simulink model "eAgriBot_V4"  (R2022b)
settings: Solver=ode3  StartTime=0.0  StopTime=t_sim  FixedStep=step_size  RelTol=1e-3
values from neighbouring files (symbols this model uses):
  accel = 0.1*9.81    (= 0.981)    [Run_eAgriBot_V4.m]
  B_tines = 5    [Run_eAgriBot_V4.m]
  brake_bias = 1    [Run_eAgriBot_V4.m]
  c = 6100    [Run_eAgriBot_V4.m]
  decel = 0.15*9.81    (= 1.4715)    [Run_eAgriBot_V4.m]
  decel_begin_dist = total_dist_target    (= 100)    [Run_eAgriBot_V4.m]
  drivetype = 3    [Run_eAgriBot_V4.m]
  effmap = [0.5 0.586 0.723 0.778 0.614 0.604 0.6 0.584 0.709 0.658 0.586 0.688 ... (121 elements, 11x11)]    [EM_effmap_generic.mat]
  end_delay = 4    [Run_eAgriBot_V4.m]
  F_tines = 5    [Run_eAgriBot_V4.m]
  Fb_max = m*g    (= 5101.2)    [Run_eAgriBot_V4.m]
  FT_c_x_rel = l_f    (= 0.645)    [Run_eAgriBot_V4.m]
  FT_c_z_rel = R_u-h_CoG    (= -0.2825)    [Run_eAgriBot_V4.m]
  g = 9.81    [Run_eAgriBot_V4.m]
  gb_eff = 0.98    [Run_eAgriBot_V4.m]
  ground_coh = c*ones(length(ground_points),1)    [Run_eAgriBot_V4.m]
  ground_dens = gamma_s*ones(length(ground_points),1)    [Run_eAgriBot_V4.m]
  ground_height = zeros(length(ground_points),1)    [Run_eAgriBot_V4.m]
  ground_kxy = k_xy*ones(length(ground_points),1)    [Run_eAgriBot_V4.m]
  ground_res = 0.01    [Run_eAgriBot_V4.m]
  Har_back_tip_x_rel = Har_back_top_x_rel+Har_tine_length*cos(Har_angle)    [Run_eAgriBot_V4.m]
  Har_back_tip_z_rel = abs(Hook_z_rel)-h_CoG-Har_tine_depth    [Run_eAgriBot_V4.m]
  Har_back_top_x_rel = -2.0    (= -2)    [Run_eAgriBot_V4.m]
  Har_back_top_z_rel = Har_back_tip_z_rel+Har_tine_length*sin(Har_angle)    [Run_eAgriBot_V4.m]
  Har_front_tip_x_rel = Har_front_top_x_rel+Har_tine_length*cos(Har_angle)    [Run_eAgriBot_V4.m]
  Har_front_tip_z_rel = abs(Hook_z_rel)-h_CoG-Har_tine_depth    [Run_eAgriBot_V4.m]
  Har_front_top_x_rel = -1.2    [Run_eAgriBot_V4.m]
  Har_front_top_z_rel = Har_front_tip_z_rel+Har_tine_length*sin(Har_angle)    [Run_eAgriBot_V4.m]
  Har_tine_length = 0.25    [Run_eAgriBot_V4.m]
  Har_tine_width = 0.02    [Run_eAgriBot_V4.m]
  Har_tire_rad = 0.5842/2    (= 0.2921)    [Run_eAgriBot_V4.m]
  Har_tire_x_rel = -1.5    [Run_eAgriBot_V4.m]
  Har_tire_z_rel = abs(Hook_z_rel)-h_CoG+Har_tire_rad    [Run_eAgriBot_V4.m]
  Hook_x_rel = l_f-l-0.4    (= -1.045)    [Run_eAgriBot_V4.m]
  Hook_z_rel = -0.3    [Run_eAgriBot_V4.m]
  i_front = 17.9542    [Run_eAgriBot_V4.m]
  I_gain = 0.0    (= 0)    [Run_eAgriBot_V4.m]
  i_rear = 17.9542    [Run_eAgriBot_V4.m]
  I_y = 150    [Run_eAgriBot_V4.m]
  I_y_tool = 20    [Run_eAgriBot_V4.m]
  index_init = round(FT_init_exit_x/ground_res)+1    [Run_eAgriBot_V4.m]
  init_CoG_height = h_CoG-0.001    (= 0.599)    [Run_eAgriBot_V4.m]
  init_CoG_v_z = 0    [Run_eAgriBot_V4.m]
  init_omega = 0    [Run_eAgriBot_V4.m]
  init_theta = 0    [Run_eAgriBot_V4.m]
  J_front = J_drive    (= 15)    [Run_eAgriBot_V4.m]
  J_harrow = 1    [Run_eAgriBot_V4.m]
  J_rear = J_drive    (= 15)    [Run_eAgriBot_V4.m]
  k_d = 50e2    (= 5000)    [Run_eAgriBot_V4.m]
  k_d_har = 50e2    (= 5000)    [Run_eAgriBot_V4.m]
  m = 520    [Run_eAgriBot_V4.m]
  m_tool = 200    [Run_eAgriBot_V4.m]
  main_cycle_delay = 5    [Run_eAgriBot_V4.m]
  mu = 0.35    [Run_eAgriBot_V4.m]
  omega_tool_init = 0    [Run_eAgriBot_V4.m]
  P_aux = 200    [Run_eAgriBot_V4.m]
  P_gain = 1.0    (= 1)    [Run_eAgriBot_V4.m]
  pack_Ah = 360    [Battery_data_V5_Kokam_NMC.mat]
  pack_R_charge = [0.00267222222222 0.00267222222222 0.00317777777778 0.00310555555556 0.0026 0.00281666666667 0.00332222222222 0.00353888888889 0.00325 0.00382777777778 0.00382777777778]    [Battery_data_V5_Kokam_NMC.mat]
  pack_R_discharge = [0.00267222222222 0.00267222222222 0.00317777777778 0.00310555555556 0.0026 0.00281666666667 0.00332222222222 0.00353888888889 0.00325 0.00382777777778 0.00382777777778]    [Battery_data_V5_Kokam_NMC.mat]
  pack_VOC = [54.509 52.351 50.895 49.556 48.477 47.645 47.008 46.449 45.825 44.941 44.941]    [Battery_data_V5_Kokam_NMC.mat]
  params2 = [exit_angle reso theta_m_max s_d_tol po]    [Run_eAgriBot_V4.m]
  phi = 26.6    [Run_eAgriBot_V4.m]
  pre_accel = 0.1*9.81    (= 0.981)    [Run_eAgriBot_V4.m]
  pre_decel = 0.15*9.81    (= 1.4715)    [Run_eAgriBot_V4.m]
  pre_decel_begin_dist = pre_dist_target-pre_decel_dist    (= 2.34454218631)    [Run_eAgriBot_V4.m]
  pre_vel = 5    [Run_eAgriBot_V4.m]
  r_front = R_u    (= 0.3175)    [Run_eAgriBot_V4.m]
  r_rear = R_u    (= 0.3175)    [Run_eAgriBot_V4.m]
  rho_t = gamma_s/9.81    (= 1664.01630989)    [Run_eAgriBot_V4.m]
  RT_c_x_rel = l_f-l    (= -0.645)    [Run_eAgriBot_V4.m]
  RT_c_z_rel = R_u-h_CoG    (= -0.2825)    [Run_eAgriBot_V4.m]
  s_init = 3    [Run_eAgriBot_V4.m]
  simu_max_time = cycle_total_time*4    (= 259.930519878)    [Run_eAgriBot_V4.m]
  slip_init = 0    [Run_eAgriBot_V4.m]
  slip_ub = r_rear*1.75    (= 0.555625)    [Run_eAgriBot_V4.m]
  slip_ub_har = Har_tire_rad*1.90    (= 0.55499)    [Run_eAgriBot_V4.m]
  SOC_init = 0.8    [Run_eAgriBot_V4.m]
  SOD = [0 0.1 0.2 0.3 0.4 0.5 0.6 0.7 0.8 0.9 1]    [Battery_data_V5_Kokam_NMC.mat]
  sr_lim_skid = -0.2    [Run_eAgriBot_V4.m]
  sr_lim_slip_f = 0.20-slip_trig    (= 0.18)    [Run_eAgriBot_V4.m]
  sr_lim_slip_r = 0.14-slip_trig    (= 0.12)    [Run_eAgriBot_V4.m]
  step_size = 1e-3    (= 0.001)    [Run_eAgriBot_V4.m]
  T = [80 80 75 70.5882352941 66.6666666667 63.1578947368 60 57.1428571429 54.5454545455 52.1739130435 50 48 ... (49 elements, 49x1)]    [EM_data_V4.mat]    (also in Run_eAgriBot_V4.m = 2*T)
  T_effmap = [0 8 16 24 32 40 48 56 64 72 80]    [EM_effmap_generic.mat]    (also in Run_eAgriBot_V4.m = 2*T_effmap)
  T_multi_r = 1.5    [Run_eAgriBot_V4.m]
  t_params = [c k_c k_phi phi k_xy gamma_s R_u wid c_0 c_1 c_0f c_1f n_0 n_1 k_1 k_2 k_3]    [Run_eAgriBot_V4.m]
  t_params_har = [c k_c k_phi phi k_xy gamma_s Har_tire_rad Har_tire_wid c_0 c_1 c_0f c_1f n_0 n_1 k_1 k_2 k_3]    [Run_eAgriBot_V4.m]
  theta_tool_init = 0    [Run_eAgriBot_V4.m]
  Tine_vz_damping = 0    [Run_eAgriBot_V4.m]
  Tool_x_rel = -1.3    [Run_eAgriBot_V4.m]
  Tool_z_rel = -0.08    [Run_eAgriBot_V4.m]
  v_init = 0    [Run_eAgriBot_V4.m]
  vel_max = 8    [Run_eAgriBot_V4.m]
  w = [0 75 80 85 90 95 100 105 110 115 120 125 ... (49 elements, 49x1)]    [EM_data_V4.mat]
  w_effmap = [0 31.4159265359 62.8318530718 94.2477796077 125.663706144 157.079632679 188.495559215 219.911485751 251.327412287 282.743338823 314.159265359]    [EM_effmap_generic.mat]
libraries: slpidlib x1, simulink x1
(part 2 of 4)

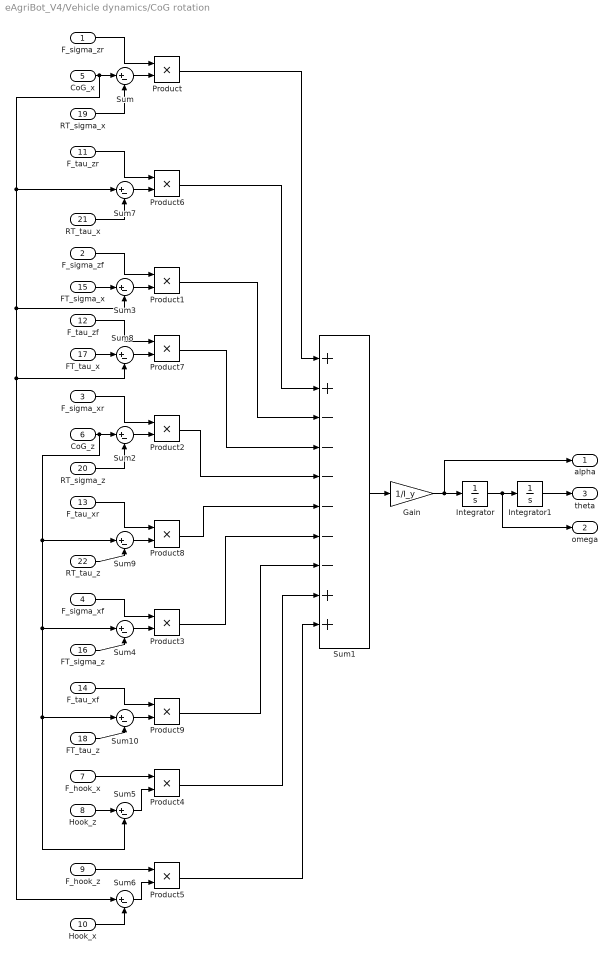
== system eAgriBot_V4/Vehicle dynamics/CoG rotation ==
  F_sigma_zr : Inport
  F_sigma_zf : Inport  Port=2
  F_sigma_xr : Inport  Port=3
  F_sigma_xf : Inport  Port=4
  CoG_x : Inport  Port=5
  CoG_z : Inport  Port=6
  F_hook_x : Inport  Port=7
  Hook_z : Inport  Port=8
  F_hook_z : Inport  Port=9
  Hook_x : Inport  Port=10
  F_tau_zr : Inport  Port=11
  F_tau_zf : Inport  Port=12
  F_tau_xr : Inport  Port=13
  F_tau_xf : Inport  Port=14
  FT_sigma_x : Inport  Port=15
  FT_sigma_z : Inport  Port=16
  FT_tau_x : Inport  Port=17
  FT_tau_z : Inport  Port=18
  RT_sigma_x : Inport  Port=19
  RT_sigma_z : Inport  Port=20
  RT_tau_x : Inport  Port=21
  RT_tau_z : Inport  Port=22
  Gain : Gain  Gain=1/I_y
  Integrator : Integrator  InitialCondition=init_omega
  Integrator1 : Integrator  InitialCondition=init_theta
  Product{,1..9} (10 alike) : Product
  Sum{,2..10} (10 alike) : Sum  Inputs=|+-
  Sum1 : Sum  Inputs=++------++
  alpha : Outport
  omega : Outport  Port=2
  theta : Outport  Port=3
  wires:
  Sum/1 -> Product/2
  F_sigma_zr/1 -> Product/1
  Product/1 -> Sum1/1
  RT_sigma_x/1 -> Sum/2
  Sum3/1 -> Product1/2
  FT_sigma_x/1 -> Sum3/1
  F_sigma_zf/1 -> Product1/1
  Sum1/1 -> Gain/1
  Integrator/1 -> omega/1, Integrator1/1
  Integrator1/1 -> theta/1
  F_sigma_xr/1 -> Product2/1
  Sum2/1 -> Product2/2
  RT_sigma_z/1 -> Sum2/2
  F_sigma_xf/1 -> Product3/1
  Sum4/1 -> Product3/2
  FT_sigma_z/1 -> Sum4/2
  Gain/1 -> alpha/1, Integrator/1
  F_hook_x/1 -> Product4/1
  Hook_z/1 -> Sum5/1
  Sum5/1 -> Product4/2
  F_hook_z/1 -> Product5/1
  Sum6/1 -> Product5/2
  Hook_x/1 -> Sum6/2
  CoG_x/1 -> Sum/1, Sum7/1, Sum6/1, Sum8/2, Sum3/2
  F_tau_zr/1 -> Product6/1
  RT_tau_x/1 -> Sum7/2
  Sum7/1 -> Product6/2
  Product1/1 -> Sum1/3
  Product6/1 -> Sum1/2
  Product2/1 -> Sum1/5
  Sum8/1 -> Product7/2
  F_tau_zf/1 -> Product7/1
  FT_tau_x/1 -> Sum8/1
  Product7/1 -> Sum1/4
  RT_tau_z/1 -> Sum9/2
  Sum9/1 -> Product8/2
  F_tau_xr/1 -> Product8/1
  CoG_z/1 -> Sum2/1, Sum9/1, Sum10/1, Sum5/2, Sum4/1
  Product3/1 -> Sum1/7
  Product8/1 -> Sum1/6
  FT_tau_z/1 -> Sum10/2
  Sum10/1 -> Product9/2
  F_tau_xf/1 -> Product9/1
  Product4/1 -> Sum1/9
  Product5/1 -> Sum1/10
  Product9/1 -> Sum1/8

== system eAgriBot_V4/Vehicle dynamics/Ground properties update for rear tire ==
  FT_x : Inport
  FT_z : Inport  Port=2
  sr_f : Inport  Port=3
  RT_x : Inport  Port=4
  RT_z : Inport  Port=5
  Constant : Constant  Value=ground_res
  Constant1 : Constant  Value=ground_res
  Constant2 : Constant  Value=params2
  Constant3 : Constant  Value=t_params
  Constant4 : Constant  Value=t_params
  Delay : Delay  DelayLength=1  InitialCondition=ground_height  SampleTime=step_size
  Delay1 : Delay  DelayLength=1  InitialCondition=index_init  SampleTime=step_size
  Delay2 : Delay  DelayLength=1  InitialCondition=ground_kxy  SampleTime=step_size
  Delay3 : Delay  DelayLength=1  InitialCondition=ground_coh  SampleTime=step_size
  Delay4 : Delay  DelayLength=1  InitialCondition=ground_dens  SampleTime=step_size
  MATLAB Function : MATLAB Function  TreatAsAtomicUnit=on  SystemSampleTime=step_size
  MATLAB Function1 : MATLAB Function  TreatAsAtomicUnit=on  SystemSampleTime=step_size
  Mux : Mux
  To Workspace : ToWorkspace  VariableName=new_gh  SampleTime=step_size
      settings: MaxDataPoints=1  Save2DSignal=2-D array (concatenate along first dimension)
  To Workspace1 : ToWorkspace  VariableName=new_dens  SampleTime=step_size
      settings: MaxDataPoints=1
  To Workspace2 : ToWorkspace  VariableName=new_coh  SampleTime=step_size
      settings: MaxDataPoints=1
  To Workspace3 : ToWorkspace  VariableName=new_kx  SampleTime=step_size
      settings: MaxDataPoints=1
  To Workspace4 : ToWorkspace  VariableName=RT_z_relative  SaveFormat=Timeseries  SampleTime=step_size
  RT_upd_params : Outport
  index_upd_high : Outport  Port=2
  index_upd_low : Outport  Port=3
  upd_h : Outport  Port=4
  upd_rho : Outport  Port=5
  upd_coh : Outport  Port=6
  upd_kx : Outport  Port=7
  wires:
  Constant/1 -> MATLAB Function/2(ground_res)
  FT_x/1 -> MATLAB Function/4(FT_x)
  FT_z/1 -> MATLAB Function/5(FT_z)
  Constant2/1 -> MATLAB Function/3(params2)
  MATLAB Function/3(ground_height) -> upd_h/1, Delay/1, To Workspace/1
  MATLAB Function/7(index) -> Delay1/1
  Delay/1 -> MATLAB Function/7("ground_height "), MATLAB Function1/3(ground_height)
  Delay1/1 -> MATLAB Function/11(prev_index)
  Constant3/1 -> MATLAB Function/1(t_params)
  sr_f/1 -> MATLAB Function/6(sr_f)
  MATLAB Function/6(kx) -> upd_kx/1, Delay2/1, To Workspace3/1
  Delay2/1 -> MATLAB Function/10("kx "), MATLAB Function1/6(kx)
  MATLAB Function/5(coh) -> upd_coh/1, Delay3/1, To Workspace2/1
  Delay3/1 -> MATLAB Function/9("coh "), MATLAB Function1/5(coh)
  MATLAB Function/4(dens) -> upd_rho/1, Delay4/1, To Workspace1/1
  Delay4/1 -> MATLAB Function/8("dens "), MATLAB Function1/4(dens)
  RT_x/1 -> MATLAB Function1/1(RT_x)
  Constant1/1 -> MATLAB Function1/7(ground_res)
  Constant4/1 -> MATLAB Function1/8(t_params)
  RT_z/1 -> MATLAB Function1/2(RT_z)
  MATLAB Function1/1(upd_RT_z) -> To Workspace4/1, Mux/1
  MATLAB Function1/2(upd_dens) -> Mux/2
  MATLAB Function1/3(upd_coh) -> Mux/3
  MATLAB Function1/4(upd_kx) -> Mux/4
  Mux/1 -> RT_upd_params/1
  MATLAB Function/1(index_upd_high) -> index_upd_high/1
  MATLAB Function/2(index_upd_low) -> index_upd_low/1

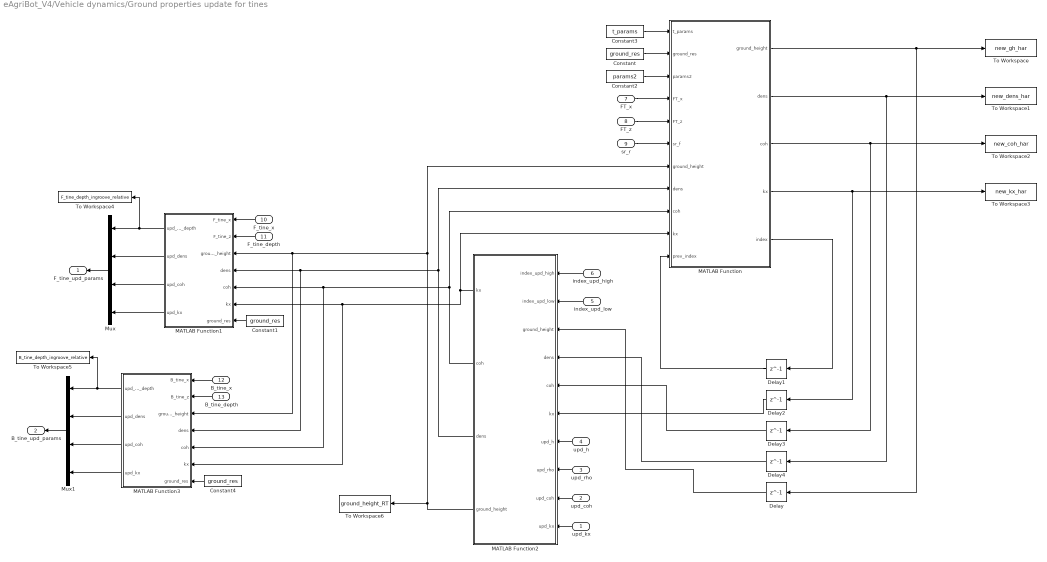
== system eAgriBot_V4/Vehicle dynamics/Ground properties update for tines ==
  upd_kx : Inport
  upd_coh : Inport  Port=2
  upd_rho : Inport  Port=3
  upd_h : Inport  Port=4
  index_upd_low : Inport  Port=5
  index_upd_high : Inport  Port=6
  FT_x : Inport  Port=7
  FT_z : Inport  Port=8
  sr_r : Inport  Port=9
  F_tine_x : Inport  Port=10
  F_tine_depth : Inport  Port=11
  B_tine_x : Inport  Port=12
  B_tine_depth : Inport  Port=13
  Constant : Constant  Value=ground_res
  Constant1 : Constant  Value=ground_res
  Constant2 : Constant  Value=params2
  Constant3 : Constant  Value=t_params
  Constant4 : Constant  Value=ground_res
  Delay : Delay  DelayLength=1  InitialCondition=ground_height  SampleTime=step_size
  Delay1 : Delay  DelayLength=1  InitialCondition=index_init  SampleTime=step_size
  Delay2 : Delay  DelayLength=1  InitialCondition=ground_kxy  SampleTime=step_size
  Delay3 : Delay  DelayLength=1  InitialCondition=ground_coh  SampleTime=step_size
  Delay4 : Delay  DelayLength=1  InitialCondition=ground_dens  SampleTime=step_size
  MATLAB Function : MATLAB Function  TreatAsAtomicUnit=on  SystemSampleTime=step_size
  MATLAB Function1 : MATLAB Function  TreatAsAtomicUnit=on  SystemSampleTime=step_size
  MATLAB Function2 : MATLAB Function  TreatAsAtomicUnit=on  SystemSampleTime=step_size
  MATLAB Function3 : MATLAB Function  TreatAsAtomicUnit=on  SystemSampleTime=step_size
  Mux : Mux
  Mux1 : Mux
  To Workspace : ToWorkspace  VariableName=new_gh_har  SampleTime=step_size
      settings: MaxDataPoints=1  Save2DSignal=2-D array (concatenate along first dimension)
  To Workspace1 : ToWorkspace  VariableName=new_dens_har  SampleTime=step_size
      settings: MaxDataPoints=1
  To Workspace2 : ToWorkspace  VariableName=new_coh_har  SampleTime=step_size
      settings: MaxDataPoints=1
  To Workspace3 : ToWorkspace  VariableName=new_kx_har  SampleTime=step_size
      settings: MaxDataPoints=1
  To Workspace4 : ToWorkspace  VariableName=F_tine_depth_ingroove_relative  SaveFormat=Timeseries  SampleTime=step_size
  To Workspace5 : ToWorkspace  VariableName=B_tine_depth_ingroove_relative  SaveFormat=Timeseries  SampleTime=step_size
  To Workspace6 : ToWorkspace  VariableName=ground_height_RT  SampleTime=-1
      settings: MaxDataPoints=1
  F_tine_upd_params : Outport
  B_tine_upd_params : Outport  Port=2
  wires:
  Constant/1 -> MATLAB Function/2(ground_res)
  FT_x/1 -> MATLAB Function/4(FT_x)
  FT_z/1 -> MATLAB Function/5(FT_z)
  Constant2/1 -> MATLAB Function/3(params2)
  MATLAB Function/1(ground_height) -> Delay/1, To Workspace/1
  MATLAB Function/5(index) -> Delay1/1
  Delay/1 -> MATLAB Function2/3("ground_height ")
  Delay1/1 -> MATLAB Function/11(prev_index)
  Constant3/1 -> MATLAB Function/1(t_params)
  sr_r/1 -> MATLAB Function/6(sr_f)
  MATLAB Function/4(kx) -> To Workspace3/1, Delay2/1
  Delay2/1 -> MATLAB Function2/6("kx ")
  MATLAB Function/3(coh) -> To Workspace2/1, Delay3/1
  Delay3/1 -> MATLAB Function2/5("coh ")
  MATLAB Function/2(dens) -> To Workspace1/1, Delay4/1
  Delay4/1 -> MATLAB Function2/4("dens ")
  F_tine_x/1 -> MATLAB Function1/1(F_tine_x)
  Constant1/1 -> MATLAB Function1/7(ground_res)
  F_tine_depth/1 -> MATLAB Function1/2(F_tine_z)
  MATLAB Function1/1(upd_F_tine_depth) -> To Workspace4/1, Mux/1
  MATLAB Function1/2(upd_dens) -> Mux/2
  MATLAB Function1/3(upd_coh) -> Mux/3
  MATLAB Function1/4(upd_kx) -> Mux/4
  Mux/1 -> F_tine_upd_params/1
  index_upd_high/1 -> MATLAB Function2/1(index_upd_high)
  index_upd_low/1 -> MATLAB Function2/2(index_upd_low)
  MATLAB Function2/4(ground_height) -> To Workspace6/1, MATLAB Function/7("ground_height "), MATLAB Function3/3(ground_height), MATLAB Function1/3(ground_height)
  MATLAB Function2/3(dens) -> MATLAB Function/8("dens "), MATLAB Function3/4(dens), MATLAB Function1/4(dens)
  MATLAB Function2/2(coh) -> MATLAB Function/9("coh "), MATLAB Function3/5(coh), MATLAB Function1/5(coh)
  MATLAB Function2/1(kx) -> MATLAB Function3/6(kx), MATLAB Function1/6(kx), MATLAB Function/10("kx ")
  Constant4/1 -> MATLAB Function3/7(ground_res)
  MATLAB Function3/1(upd_B_tine_depth) -> To Workspace5/1, Mux1/1
  Mux1/1 -> B_tine_upd_params/1
  MATLAB Function3/4(upd_kx) -> Mux1/4
  B_tine_depth/1 -> MATLAB Function3/2(B_tine_z)
  B_tine_x/1 -> MATLAB Function3/1(B_tine_x)
  MATLAB Function3/2(upd_dens) -> Mux1/2
  MATLAB Function3/3(upd_coh) -> Mux1/3
  upd_h/1 -> MATLAB Function2/7(upd_h)
  upd_rho/1 -> MATLAB Function2/8(upd_rho)
  upd_coh/1 -> MATLAB Function2/9(upd_coh)
  upd_kx/1 -> MATLAB Function2/10(upd_kx)

== system eAgriBot_V4/Vehicle dynamics/Position and velocity of the wheels (output values are for wheel bottom points) ==
  theta : Inport
  omega : Inport  Port=2
  CoG_vx : Inport  Port=3
  CoG_x : Inport  Port=4
  CoG_vz : Inport  Port=5
  CoG_z : Inport  Port=6
  F_sigma_anglef : Inport  Port=7
  F_tau_anglef : Inport  Port=8
  F_sigma_angler : Inport  Port=9
  F_tau_angler : Inport  Port=10
  Constant : Constant  Value=RT_c_z_rel
  Constant1 : Constant  Value=RT_c_x_rel
  Constant2 : Constant  Value=FT_c_z_rel
  Constant3 : Constant  Value=FT_c_x_rel
  Constant4 : Constant  Value=r_rear
  Constant5 : Constant  Value=r_front
  MATLAB Function : MATLAB Function  TreatAsAtomicUnit=on  SystemSampleTime=step_size
  MATLAB Function1 : MATLAB Function  TreatAsAtomicUnit=on  SystemSampleTime=step_size
  RT_x : Outport
  RT_z : Outport  Port=2
  FT_x : Outport  Port=3
  FT_z : Outport  Port=4
  RT_vx : Outport  Port=5
  RT_vz : Outport  Port=6
  FT_vx : Outport  Port=7
  FT_vz : Outport  Port=8
  FT_sigma_x : Outport  Port=9
  FT_sigma_z : Outport  Port=10
  FT_tau_x : Outport  Port=11
  FT_tau_z : Outport  Port=12
  RT_sigma_x : Outport  Port=13
  RT_sigma_z : Outport  Port=14
  RT_tau_x : Outport  Port=15
  RT_tau_z : Outport  Port=16
  wires:
  MATLAB Function/4(FT_z) -> MATLAB Function1/4(FT_z), FT_z/1
  MATLAB Function/8(FT_vz) -> FT_vz/1
  CoG_vz/1 -> MATLAB Function/5(CoG_vz)
  theta/1 -> MATLAB Function/1(theta)
  CoG_vx/1 -> MATLAB Function/3(CoG_vx)
  MATLAB Function/1(RT_x) -> MATLAB Function1/1(RT_x), RT_x/1
  omega/1 -> MATLAB Function/2(omega)
  MATLAB Function/6(RT_vz) -> RT_vz/1
  MATLAB Function/3(FT_x) -> MATLAB Function1/3(FT_x), FT_x/1
  MATLAB Function/7(FT_vx) -> FT_vx/1
  MATLAB Function/5(RT_vx) -> RT_vx/1
  CoG_z/1 -> MATLAB Function/6(CoG_z)
  CoG_x/1 -> MATLAB Function/4(CoG_x)
  MATLAB Function/2(RT_z) -> MATLAB Function1/2(RT_z), RT_z/1
  Constant/1 -> MATLAB Function/7(RT_c_z_rel)
  Constant1/1 -> MATLAB Function/8(RT_c_x_rel)
  Constant2/1 -> MATLAB Function/9(FT_c_z_rel)
  Constant3/1 -> MATLAB Function/10(FT_c_x_rel)
  Constant4/1 -> MATLAB Function1/5(r_rear), MATLAB Function/11(r_rear)
  Constant5/1 -> MATLAB Function/12(r_front), MATLAB Function1/6(r_front)
  MATLAB Function1/1(FT_sigma_x) -> FT_sigma_x/1
  MATLAB Function1/2(FT_sigma_z) -> FT_sigma_z/1
  MATLAB Function1/3(FT_tau_x) -> FT_tau_x/1
  MATLAB Function1/4(FT_tau_z) -> FT_tau_z/1
  MATLAB Function1/5(RT_sigma_x) -> RT_sigma_x/1
  MATLAB Function1/6(RT_sigma_z) -> RT_sigma_z/1
  MATLAB Function1/7(RT_tau_x) -> RT_tau_x/1
  MATLAB Function1/8(RT_tau_z) -> RT_tau_z/1
  F_sigma_anglef/1 -> MATLAB Function1/7(F_sigma_anglef)
  F_tau_anglef/1 -> MATLAB Function1/8(F_tau_anglef)
  F_sigma_angler/1 -> MATLAB Function1/9(F_sigma_angler)
  F_tau_angler/1 -> MATLAB Function1/10(F_tau_angler)

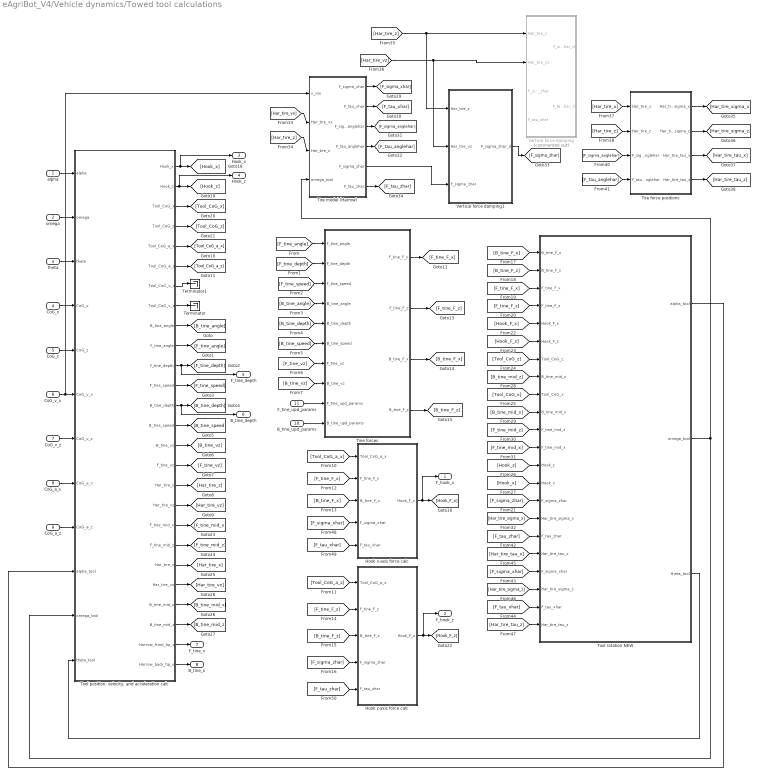
== system eAgriBot_V4/Vehicle dynamics/Towed tool calculations ==
  alpha : Inport
  omega : Inport  Port=2
  theta : Inport  Port=3
  CoG_x : Inport  Port=4
  CoG_z : Inport  Port=5
  CoG_v_x : Inport  Port=6
  CoG_v_z : Inport  Port=7
  CoG_a_x : Inport  Port=8
  CoG_a_z : Inport  Port=9
  B_tine_upd_params : Inport  Port=10
  F_tine_upd_params : Inport  Port=11
  Hook x-axis force calc : Subsystem
      settings: MinAlgLoopOccurrences=on
  Hook z-axis force calc : Subsystem
      settings: MinAlgLoopOccurrences=on
  Terminator : Terminator
  Terminator1 : Terminator
  Tine forces : Subsystem
  Tire force positions : Subsystem
  Tire model (Harrow) : Subsystem
  "Tool position, velocity, and acceleration calc" : Subsystem
      settings: MinAlgLoopOccurrences=on
  Tool rotation NEW : Subsystem
  Vertical force damping : Subsystem  Commented=on
  Vertical force damping1 : Subsystem
  F_hook_x : Outport
  F_hook_z : Outport  Port=2
  Hook_x : Outport  Port=3
  Hook_z : Outport  Port=4
  F_tine_depth : Outport  Port=5
  B_tine_depth : Outport  Port=6
  F_tine_x : Outport  Port=7
  B_tine_x : Outport  Port=8
  wires:
  alpha/1 -> "Tool position, velocity, and acceleration calc"/1(alpha)
  omega/1 -> "Tool position, velocity, and acceleration calc"/2(omega)
  theta/1 -> "Tool position, velocity, and acceleration calc"/3(theta)
  CoG_x/1 -> "Tool position, velocity, and acceleration calc"/4(CoG_x)
  CoG_z/1 -> "Tool position, velocity, and acceleration calc"/5(CoG_z)
  CoG_v_x/1 -> Tire model (Harrow)/1(v_ms), "Tool position, velocity, and acceleration calc"/6(CoG_v_x)
  CoG_v_z/1 -> "Tool position, velocity, and acceleration calc"/7(CoG_v_z)
  Hook x-axis force calc/1(Hook_F_x) -> F_hook_x/1, [Hook_F_x]
  CoG_a_x/1 -> "Tool position, velocity, and acceleration calc"/8(CoG_a_x)
  CoG_a_z/1 -> "Tool position, velocity, and acceleration calc"/9(CoG_a_z)
  Tool rotation NEW/3(theta_tool) -> "Tool position, velocity, and acceleration calc"/12(theta_tool)
  Tool rotation NEW/2(omega_tool) -> Tire model (Harrow)/4(omega_tool), "Tool position, velocity, and acceleration calc"/11(omega_tool)
  "Tool position, velocity, and acceleration calc"/9(B_tine_angle) -> [B_tine_angle]
  "Tool position, velocity, and acceleration calc"/10(F_tine_angle) -> [F_tine_angle]
  "Tool position, velocity, and acceleration calc"/11(F_tine_depth) -> F_tine_depth/1, [F_tine_depth]
  "Tool position, velocity, and acceleration calc"/12(F_tine_speed) -> [F_tine_speed]
  "Tool position, velocity, and acceleration calc"/13(B_tine_depth) -> B_tine_depth/1, [B_tine_depth]
  "Tool position, velocity, and acceleration calc"/14(B_tine_speed) -> [B_tine_speed]
  [F_tine_angle] -> Tine forces/1(F_tine_angle)
  [B_tine_speed] -> Tine forces/6(B_tine_speed)
  [B_tine_depth] -> Tine forces/5(B_tine_depth)
  [B_tine_angle] -> Tine forces/4(B_tine_angle)
  [F_tine_speed] -> Tine forces/3(F_tine_speed)
  [F_tine_depth] -> Tine forces/2(F_tine_depth)
  "Tool position, velocity, and acceleration calc"/15(B_tine_vz) -> [B_tine_vz]
  "Tool position, velocity, and acceleration calc"/16(F_tine_vz) -> [F_tine_vz]
  [F_tine_vz] -> Tine forces/7(F_tine_vz)
  [B_tine_vz] -> Tine forces/8(B_tine_vz)
  "Tool position, velocity, and acceleration calc"/17(Har_tire_z) -> [Har_tire_z]
  "Tool position, velocity, and acceleration calc"/18(Har_tire_vz) -> [Har_tire_vz]
  "Tool position, velocity, and acceleration calc"/5(Tool_CoG_a_x) -> [Tool_CoG_a_x]
  [Tool_CoG_a_x] -> Hook x-axis force calc/1(Tool_CoG_a_x)
  "Tool position, velocity, and acceleration calc"/6(Tool_CoG_a_z) -> [Tool_CoG_a_z]
  [Tool_CoG_a_z] -> Hook z-axis force calc/1(Tool_CoG_a_z)
  Tine forces/1(F_tine_F_x) -> [F_tine_F_x]
  Tine forces/2(F_tine_F_z) -> [F_tine_F_z]
  Tine forces/3(B_tine_F_x) -> [B_tine_F_x]
  Tine forces/4(B_tine_F_z) -> [B_tine_F_z]
  [F_tine_F_x] -> Hook x-axis force calc/2(F_tine_F_x)
  [B_tine_F_x] -> Hook x-axis force calc/3(B_tine_F_x)
  [F_tine_F_z] -> Hook z-axis force calc/2(F_tine_F_z)
  [B_tine_F_z] -> Hook z-axis force calc/3(B_tine_F_z)
  "Tool position, velocity, and acceleration calc"/1(Hook_x) -> Hook_x/1, [Hook_x]
  "Tool position, velocity, and acceleration calc"/2(Hook_z) -> Hook_z/1, [Hook_z]
  "Tool position, velocity, and acceleration calc"/3(Tool_CoG_x) -> [Tool_CoG_x]
  "Tool position, velocity, and acceleration calc"/4(Tool_CoG_z) -> [Tool_CoG_z]
  Hook z-axis force calc/1(Hook_F_z) -> F_hook_z/1, [Hook_F_z]
  [B_tine_F_x] -> Tool rotation NEW/1(B_tine_F_x)
  [B_tine_F_z] -> Tool rotation NEW/2(B_tine_F_z)
  [F_tine_F_x] -> Tool rotation NEW/3(F_tine_F_x)
  [F_tine_F_z] -> Tool rotation NEW/4(F_tine_F_z)
  [F_sigma_zhar] -> Tool rotation NEW/15(F_sigma_zhar)
  [Hook_F_x] -> Tool rotation NEW/5(Hook_F_x)
  [Hook_F_z] -> Tool rotation NEW/6(Hook_F_z)
  [Tool_CoG_z] -> Tool rotation NEW/7(Tool_CoG_z)
  [Tool_CoG_x] -> Tool rotation NEW/9(Tool_CoG_x)
  [Hook_z] -> Tool rotation NEW/13(Hook_z)
  [Hook_x] -> Tool rotation NEW/14(Hook_x)
  "Tool position, velocity, and acceleration calc"/19(F_tine_mid_x) -> [F_tine_mid_x]
  "Tool position, velocity, and acceleration calc"/20(F_tine_mid_z) -> [F_tine_mid_z]
  "Tool position, velocity, and acceleration calc"/21(Har_tire_x) -> [Har_tire_x]
  "Tool position, velocity, and acceleration calc"/23(B_tine_mid_x) -> [B_tine_mid_x]
  "Tool position, velocity, and acceleration calc"/24(B_tine_mid_z) -> [B_tine_mid_z]
  [B_tine_mid_z] -> Tool rotation NEW/8(B_tine_mid_z)
  [B_tine_mid_x] -> Tool rotation NEW/10(B_tine_mid_x)
  [F_tine_mid_z] -> Tool rotation NEW/11(F_tine_mid_z)
  [F_tine_mid_x] -> Tool rotation NEW/12(F_tine_mid_x)
  [Har_tire_sigma_x] -> Tool rotation NEW/16(Har_tire_sigma_x)
  "Tool position, velocity, and acceleration calc"/22(Har_tire_vx) -> [Har_tire_vx]
  [Har_tire_vx] -> Tire model (Harrow)/2(Har_tire_vx)
  [Har_tire_z] -> Tire model (Harrow)/3(Har_tire_z)
  [Har_tire_z] -> Vertical force damping1/1(Har_tire_z), Vertical force damping/1(Har_tire_z)
  [Har_tire_vz] -> Vertical force damping1/2(Har_tire_vz), Vertical force damping/2(Har_tire_vz)
  Tire model (Harrow)/1(F_sigma_xhar) -> [F_sigma_xhar]
  Tire model (Harrow)/2(F_tau_xhar) -> [F_tau_xhar]
  Tire model (Harrow)/3(F_sigma_anglehar) -> [F_sigma_anglehar]
  Tire model (Harrow)/4(F_tau_anglehar) -> [F_tau_anglehar]
  [F_tau_zhar] -> Tool rotation NEW/17(F_tau_zhar)
  [F_sigma_xhar] -> Tool rotation NEW/19(F_sigma_xhar)
  [F_tau_xhar] -> Tool rotation NEW/21(F_tau_xhar)
  [Har_tire_tau_x] -> Tool rotation NEW/18(Har_tire_tau_x)
  [Har_tire_sigma_z] -> Tool rotation NEW/20(Har_tire_sigma_z)
  [Har_tire_tau_z] -> Tool rotation NEW/22(Har_tire_tau_z)
  [F_sigma_xhar] -> Hook x-axis force calc/4(F_sigma_xhar)
  [F_tau_xhar] -> Hook x-axis force calc/5(F_tau_xhar)
  [F_sigma_zhar] -> Hook z-axis force calc/4(F_sigma_zhar)
  [F_tau_zhar] -> Hook z-axis force calc/5(F_tau_zhar)
  [Har_tire_x] -> Tire force positions/1(Har_tire_x)
  [Har_tire_z] -> Tire force positions/2(Har_tire_z)
  [F_sigma_anglehar] -> Tire force positions/3(F_sigma_anglehar)
  [F_tau_anglehar] -> Tire force positions/4(F_tau_anglehar)
  Tire force positions/1(Har_tire_sigma_x) -> [Har_tire_sigma_x]
  Tire force positions/2(Har_tire_sigma_z) -> [Har_tire_sigma_z]
  Tire force positions/3(Har_tire_tau_x) -> [Har_tire_tau_x]
  Tire force positions/4(Har_tire_tau_z) -> [Har_tire_tau_z]
  Tool rotation NEW/1(alpha_tool) -> "Tool position, velocity, and acceleration calc"/10(alpha_tool)
  Tire model (Harrow)/6(F_tau_zhar) -> [F_tau_zhar]
  Tire model (Harrow)/5(F_sigma_zhar) -> Vertical force damping1/3(F_sigma_zhar)
  Vertical force damping1/1(F_sigma_zhar_d) -> [F_sigma_zhar]
  "Tool position, velocity, and acceleration calc"/7(Tool_CoG_v_x) -> Terminator1/1
  "Tool position, velocity, and acceleration calc"/8(Tool_CoG_v_z) -> Terminator/1
  "Tool position, velocity, and acceleration calc"/25(Harrow_front_tip_x) -> F_tine_x/1
  "Tool position, velocity, and acceleration calc"/26(Harrow_back_tip_x) -> B_tine_x/1
  F_tine_upd_params/1 -> Tine forces/9(F_tine_upd_params)
  B_tine_upd_params/1 -> Tine forces/10(B_tine_upd_params)

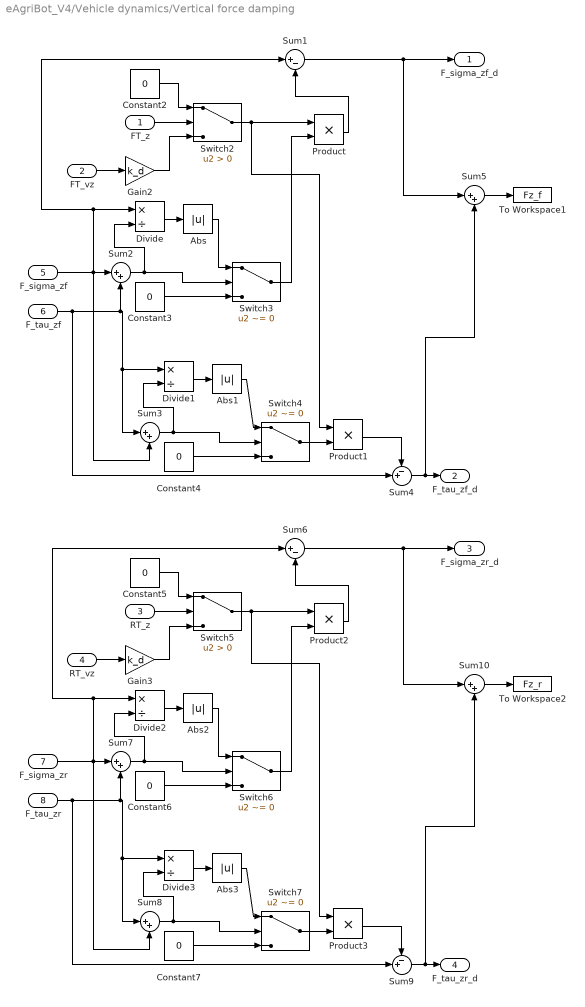
== system eAgriBot_V4/Vehicle dynamics/Vertical force damping ==
  FT_z : Inport
  FT_vz : Inport  Port=2
  RT_z : Inport  Port=3
  RT_vz : Inport  Port=4
  F_sigma_zf : Inport  Port=5
  F_tau_zf : Inport  Port=6
  F_sigma_zr : Inport  Port=7
  F_tau_zr : Inport  Port=8
  Abs{,1..3} (4 alike) : Abs  SaturateOnIntegerOverflow=off
  Constant{2..7} (6 alike) : Constant  Value=0
  Divide{,1..3} (4 alike) : Product  Inputs=*/
  Gain2 : Gain  Gain=k_d
  Gain3 : Gain  Gain=k_d
  Product{,1..3} (4 alike) : Product
  Sum1 : Sum  Inputs=|+-
  Sum{2..3,5,7..8,10} (6 alike) : Sum  Inputs=|++
  Sum4 : Sum  Inputs=-+|
  Sum6 : Sum  Inputs=|+-
  Sum9 : Sum  Inputs=-+|
  Switch2 : Switch  Criteria=u2 > Threshold  SaturateOnIntegerOverflow=off  InputSameDT=off
  Switch{3..4,6..7} (4 alike) : Switch  Criteria=u2 ~= 0  SaturateOnIntegerOverflow=off  InputSameDT=off
  Switch5 : Switch  Criteria=u2 > Threshold  SaturateOnIntegerOverflow=off  InputSameDT=off
  To Workspace1 : ToWorkspace  VariableName=Fz_f  SaveFormat=Timeseries  SampleTime=-1
  To Workspace2 : ToWorkspace  VariableName=Fz_r  SaveFormat=Timeseries  SampleTime=-1
  F_sigma_zf_d : Outport
  F_tau_zf_d : Outport  Port=2
  F_sigma_zr_d : Outport  Port=3
  F_tau_zr_d : Outport  Port=4
  wires:
  Sum1/1 -> Sum5/1, F_sigma_zf_d/1
  FT_vz/1 -> Gain2/1
  Gain2/1 -> Switch2/3
  FT_z/1 -> Switch2/2
  Switch2/1 -> Product1/1, Product/1
  Constant2/1 -> Switch2/1
  Sum2/1 -> Divide/2, Switch3/2
  Constant3/1 -> Switch3/3
  Divide/1 -> Abs/1
  Abs/1 -> Switch3/1
  Switch3/1 -> Product/2
  Product/1 -> Sum1/2
  Sum3/1 -> Divide1/2, Switch4/2
  Abs1/1 -> Switch4/1
  Constant4/1 -> Switch4/3
  F_tau_zf/1 -> Sum4/2, Sum3/1, Divide1/1, Sum2/2
  Divide1/1 -> Abs1/1
  F_sigma_zf/1 -> Sum2/1, Sum3/2, Sum1/1, Divide/1
  Switch4/1 -> Product1/2
  Product1/1 -> Sum4/1
  Sum4/1 -> Sum5/2, F_tau_zf_d/1
  Sum5/1 -> To Workspace1/1
  Product3/1 -> Sum9/1
  Sum7/1 -> Divide2/2, Switch6/2
  Abs3/1 -> Switch7/1
  Sum8/1 -> Divide3/2, Switch7/2
  Constant7/1 -> Switch7/3
  Divide2/1 -> Abs2/1
  F_sigma_zr/1 -> Sum7/1, Sum8/2, Sum6/1, Divide2/1
  Sum9/1 -> Sum10/2, F_tau_zr_d/1
  Divide3/1 -> Abs3/1
  RT_z/1 -> Switch5/2
  Abs2/1 -> Switch6/1
  Constant6/1 -> Switch6/3
  RT_vz/1 -> Gain3/1
  Constant5/1 -> Switch5/1
  Sum6/1 -> Sum10/1, F_sigma_zr_d/1
  Switch6/1 -> Product2/2
  F_tau_zr/1 -> Sum9/2, Sum8/1, Divide3/1, Sum7/2
  Gain3/1 -> Switch5/3
  Switch7/1 -> Product3/2
  Switch5/1 -> Product3/1, Product2/1
  Product2/1 -> Sum6/2
  Sum10/1 -> To Workspace2/1

== system eAgriBot_V4/Vehicle dynamics/Towed tool calculations/Hook x-axis force calc ==
  Tool_CoG_a_x : Inport
  F_tine_F_x : Inport  Port=2
  B_tine_F_x : Inport  Port=3
  F_sigma_xhar : Inport  Port=4
  F_tau_xhar : Inport  Port=5
  Gain : Gain  Gain=m_tool
  Sum : Sum  Inputs=+---
  Sum1 : Sum  Inputs=|++
  To Workspace : ToWorkspace  VariableName=Tines_Fx  SaveFormat=Timeseries  SampleTime=-1
  To Workspace1 : ToWorkspace  VariableName=F_tine_Fx  SaveFormat=Timeseries  SampleTime=-1
  To Workspace2 : ToWorkspace  VariableName=B_tine_Fx  SaveFormat=Timeseries  SampleTime=-1
  Hook_F_x : Outport
  wires:
  Tool_CoG_a_x/1 -> Gain/1
  Sum/1 -> Hook_F_x/1
  Sum1/1 -> Sum/4, To Workspace/1
  B_tine_F_x/1 -> To Workspace2/1, Sum1/2
  F_tine_F_x/1 -> To Workspace1/1, Sum1/1
  F_tau_xhar/1 -> Sum/3
  F_sigma_xhar/1 -> Sum/2
  Gain/1 -> Sum/1

== system eAgriBot_V4/Vehicle dynamics/Towed tool calculations/Hook z-axis force calc ==
  Tool_CoG_a_z : Inport
  F_tine_F_z : Inport  Port=2
  B_tine_F_z : Inport  Port=3
  F_sigma_zhar : Inport  Port=4
  F_tau_zhar : Inport  Port=5
  Constant : Constant  Value=m_tool*g
  Gain : Gain  Gain=m_tool
  Sum : Sum  Inputs=++---
  Sum2 : Sum  Inputs=|++
  To Workspace : ToWorkspace  VariableName=Tines_Fz  SaveFormat=Timeseries  SampleTime=-1
  To Workspace1 : ToWorkspace  VariableName=F_tine_Fz  SaveFormat=Timeseries  SampleTime=-1
  To Workspace2 : ToWorkspace  VariableName=B_tine_Fz  SaveFormat=Timeseries  SampleTime=-1
  Hook_F_z : Outport
  wires:
  Tool_CoG_a_z/1 -> Gain/1
  Sum/1 -> Hook_F_z/1
  F_tine_F_z/1 -> To Workspace1/1, Sum2/1
  B_tine_F_z/1 -> To Workspace2/1, Sum2/2
  Sum2/1 -> Sum/5, To Workspace/1
  F_tau_zhar/1 -> Sum/4
  F_sigma_zhar/1 -> Sum/3
  Gain/1 -> Sum/2
  Constant/1 -> Sum/1

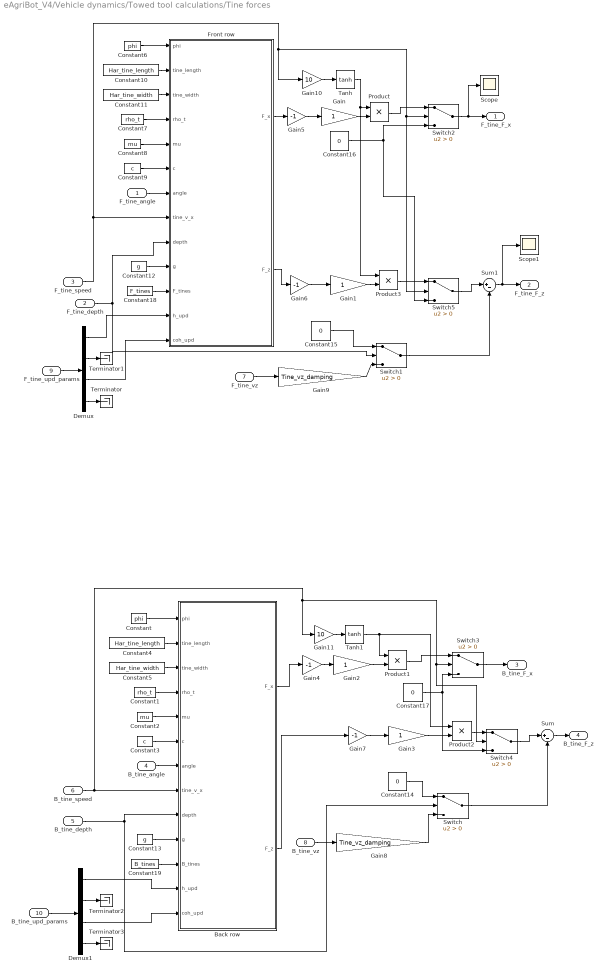
== system eAgriBot_V4/Vehicle dynamics/Towed tool calculations/Tine forces ==
  F_tine_angle : Inport
  F_tine_depth : Inport  Port=2
  F_tine_speed : Inport  Port=3
  B_tine_angle : Inport  Port=4
  B_tine_depth : Inport  Port=5
  B_tine_speed : Inport  Port=6
  F_tine_vz : Inport  Port=7
  B_tine_vz : Inport  Port=8
  F_tine_upd_params : Inport  Port=9
  B_tine_upd_params : Inport  Port=10
  Back row : MATLAB Function  TreatAsAtomicUnit=on
  Constant : Constant  Value=phi
  Constant1 : Constant  Value=rho_t
  Constant10 : Constant  Value=Har_tine_length
  Constant11 : Constant  Value=Har_tine_width
  Constant12 : Constant  Value=g
  Constant13 : Constant  Value=g
  Constant{14..17} (4 alike) : Constant  Value=0
  Constant18 : Constant  Value=F_tines
  Constant19 : Constant  Value=B_tines
  Constant2 : Constant  Value=mu
  Constant3 : Constant  Value=c
  Constant4 : Constant  Value=Har_tine_length
  Constant5 : Constant  Value=Har_tine_width
  Constant6 : Constant  Value=phi
  Constant7 : Constant  Value=rho_t
  Constant8 : Constant  Value=mu
  Constant9 : Constant  Value=c
  Demux : Demux
  Demux1 : Demux
  Front row : MATLAB Function  TreatAsAtomicUnit=on
  Gain{,1..3} (4 alike) : Gain
  Gain10 : Gain  Gain=10
  Gain11 : Gain  Gain=10
  Gain{4..7} (4 alike) : Gain  Gain=-1
  Gain8 : Gain  Gain=Tine_vz_damping
  Gain9 : Gain  Gain=Tine_vz_damping
  Product{,1..3} (4 alike) : Product
  Scope : Scope
  Scope1 : Scope
  Sum : Sum  Inputs=|+-
  Sum1 : Sum  Inputs=|+-
  Switch{,1..5} (6 alike) : Switch  Criteria=u2 > Threshold  SaturateOnIntegerOverflow=off  InputSameDT=off
  Tanh : Trigonometry  Operator=tanh
  Tanh1 : Trigonometry  Operator=tanh
  Terminator{,1..3} (4 alike) : Terminator
  F_tine_F_x : Outport
  F_tine_F_z : Outport  Port=2
  B_tine_F_x : Outport  Port=3
  B_tine_F_z : Outport  Port=4
  wires:
  Constant/1 -> Back row/1(phi)
  Constant1/1 -> Back row/4(rho_t)
  Constant2/1 -> Back row/5(mu)
  Constant3/1 -> Back row/6(c)
  Constant4/1 -> Back row/2(tine_length)
  Constant5/1 -> Back row/3(tine_width)
  Constant6/1 -> Front row/1(phi)
  Constant10/1 -> Front row/2(tine_length)
  Constant8/1 -> Front row/5(mu)
  Constant11/1 -> Front row/3(tine_width)
  Constant7/1 -> Front row/4(rho_t)
  Constant9/1 -> Front row/6(c)
  F_tine_angle/1 -> Front row/7(angle)
  F_tine_speed/1 -> Gain10/1, Switch5/2, Switch2/2, Front row/8(tine_v_x)
  B_tine_angle/1 -> Back row/7(angle)
  B_tine_depth/1 -> Back row/9(depth), Switch/2
  B_tine_speed/1 -> Back row/8(tine_v_x), Gain11/1, Switch4/2, Switch3/2
  Front row/1(F_x) -> Gain5/1
  Front row/2(F_z) -> Gain6/1
  Back row/1(F_x) -> Gain4/1
  Back row/2(F_z) -> Gain7/1
  Constant12/1 -> Front row/10(g)
  Constant13/1 -> Back row/10(g)
  Gain4/1 -> Gain2/1
  Gain5/1 -> Gain/1
  Gain6/1 -> Gain1/1
  Gain7/1 -> Gain3/1
  B_tine_vz/1 -> Gain8/1
  Sum/1 -> B_tine_F_z/1
  Gain8/1 -> Switch/3
  Constant14/1 -> Switch/1
  Switch/1 -> Sum/2
  Constant15/1 -> Switch1/1
  F_tine_vz/1 -> Gain9/1
  Gain9/1 -> Switch1/3
  Switch1/1 -> Sum1/2
  Sum1/1 -> Scope1/1, F_tine_F_z/1
  F_tine_depth/1 -> Switch1/2, Front row/9(depth)
  Constant16/1 -> Switch5/3, Switch2/3
  Gain/1 -> Product/2
  Gain10/1 -> Tanh/1
  Tanh/1 -> Product3/1, Product/1
  Product/1 -> Switch2/1
  Switch2/1 -> Scope/1, F_tine_F_x/1
  Constant17/1 -> Switch3/3, Switch4/3
  Gain2/1 -> Product1/2
  Gain11/1 -> Tanh1/1
  Tanh1/1 -> Product2/1, Product1/1
  Product1/1 -> Switch3/1
  Switch3/1 -> B_tine_F_x/1
  F_tine_upd_params/1 -> Demux/1
  Demux/1 -> Front row/12(h_upd)
  Demux/3 -> Front row/13(coh_upd)
  Demux/4 -> Terminator/1
  Constant18/1 -> Front row/11(F_tines)
  Demux/2 -> Terminator1/1
  B_tine_upd_params/1 -> Demux1/1
  Demux1/1 -> Back row/12(h_upd)
  Demux1/3 -> Back row/13(coh_upd)
  Demux1/2 -> Terminator2/1
  Demux1/4 -> Terminator3/1
  Constant19/1 -> Back row/11(B_tines)
  Gain3/1 -> Product2/2
  Product2/1 -> Switch4/1
  Switch4/1 -> Sum/1
  Gain1/1 -> Product3/2
  Product3/1 -> Switch5/1
  Switch5/1 -> Sum1/1

== system eAgriBot_V4/Vehicle dynamics/Towed tool calculations/Tire force positions ==
  Har_tire_x : Inport
  Har_tire_z : Inport  Port=2
  F_sigma_anglehar : Inport  Port=3
  F_tau_anglehar : Inport  Port=4
  Constant : Constant  Value=Har_tire_rad
  MATLAB Function1 : MATLAB Function  TreatAsAtomicUnit=on  SystemSampleTime=step_size
  Har_tire_sigma_x : Outport
  Har_tire_sigma_z : Outport  Port=2
  Har_tire_tau_x : Outport  Port=3
  Har_tire_tau_z : Outport  Port=4
  wires:
  MATLAB Function1/4(Har_tire_tau_z) -> Har_tire_tau_z/1
  MATLAB Function1/2(Har_tire_sigma_z) -> Har_tire_sigma_z/1
  MATLAB Function1/1(Har_tire_sigma_x) -> Har_tire_sigma_x/1
  Har_tire_x/1 -> MATLAB Function1/1(Har_tire_x)
  F_tau_anglehar/1 -> MATLAB Function1/5(F_tau_anglehar)
  F_sigma_anglehar/1 -> MATLAB Function1/4(F_sigma_anglehar)
  Constant/1 -> MATLAB Function1/3(Har_tire_rad)
  Har_tire_z/1 -> MATLAB Function1/2(Har_tire_z)
  MATLAB Function1/3(Har_tire_tau_x) -> Har_tire_tau_x/1

== system eAgriBot_V4/Vehicle dynamics/Towed tool calculations/Tire model (Harrow) ==
  v_ms : Inport
  Har_tire_vx : Inport  Port=2
  Har_tire_z : Inport  Port=3
  omega_tool : Inport  Port=4
  1/J : Gain  Gain=1/J_harrow
  Constant : Constant  Value=slip_ub_har
  Constant1 : Constant  Value=0
  Constant2 : Constant  Value=t_params_har
  Constant3 : Constant  Value=params2
  Gain{2..6} (5 alike) : Gain  Gain=2
  Gain7 : Gain  Gain=Har_tire_rad
  Integrator : Integrator  InitialCondition=v_init/r_rear*(1+slip_init)  LimitOutput=on  LowerSaturationLimit=0
  Sum : Sum  Inputs=+-
  Sum1 : Sum  Inputs=|++
  Sum2 : Sum  Inputs=|++
  Tire force calc1 : MATLAB Function  TreatAsAtomicUnit=on  SystemSampleTime=step_size
  To Workspace : ToWorkspace  VariableName=T_Ft_har  SaveFormat=Timeseries  SampleTime=-1
  To Workspace1 : ToWorkspace  VariableName=SR_har  SaveFormat=Timeseries  SampleTime=-1
  To Workspace2 : ToWorkspace  VariableName=w_tire_har  SaveFormat=Timeseries  SampleTime=-1
  To Workspace3 : ToWorkspace  VariableName=F_sigma_anglehar  SaveFormat=Timeseries  SampleTime=-1
  To Workspace4 : ToWorkspace  VariableName=T_Ft_res_har  SaveFormat=Timeseries  SampleTime=-1
  To Workspace5 : ToWorkspace  VariableName=F_tau_anglehar  SaveFormat=Timeseries  SampleTime=-1
  r : Constant  Value=Har_tire_rad
  slip_ratio calc : MATLAB Function  TreatAsAtomicUnit=on  SystemSampleTime=step_size
  F_sigma_xhar : Outport
  F_tau_xhar : Outport  Port=2
  F_sigma_anglehar : Outport  Port=3
  F_tau_anglehar : Outport  Port=4
  F_sigma_zhar : Outport  Port=5
  F_tau_zhar : Outport  Port=6
  wires:
  1/J/1 -> Integrator/1
  Sum/1 -> 1/J/1
  Constant1/1 -> Sum/1
  v_ms/1 -> Tire force calc1/1(v_ms), slip_ratio calc/2(v_ms)
  slip_ratio calc/1(sr) -> Tire force calc1/2(s_d), To Workspace1/1
  Integrator/1 -> To Workspace2/1, Sum1/1, Tire force calc1/6(w_tire_pure)
  Tire force calc1/2(F_sigma_z) -> Gain3/1
  Har_tire_vx/1 -> slip_ratio calc/3(Har_tire_vx)
  r/1 -> slip_ratio calc/1(r_har)
  Tire force calc1/3(F_sigma_x) -> Gain4/1
  Sum1/1 -> slip_ratio calc/4(w_tire)
  Har_tire_z/1 -> Tire force calc1/3(h)
  Constant2/1 -> Tire force calc1/4(t_params)
  Constant3/1 -> Tire force calc1/5(params2)
  Gain2/1 -> To Workspace4/1, Sum/2
  Gain3/1 -> F_sigma_zhar/1
  Tire force calc1/4(F_sigma_angle) -> F_sigma_anglehar/1, To Workspace3/1
  Tire force calc1/5(F_tau_z) -> Gain5/1
  Gain5/1 -> F_tau_zhar/1
  Tire force calc1/6(F_tau_x) -> Gain6/1
  Tire force calc1/7(F_tau_angle) -> F_tau_anglehar/1, To Workspace5/1
  Sum2/1 -> Gain7/1
  Gain7/1 -> To Workspace/1
  Gain4/1 -> Sum2/1, F_sigma_xhar/1
  Gain6/1 -> F_tau_xhar/1, Sum2/2
  Tire force calc1/1(T) -> Gain2/1
  Constant/1 -> slip_ratio calc/5(slip_ub_har)
  omega_tool/1 -> Sum1/2

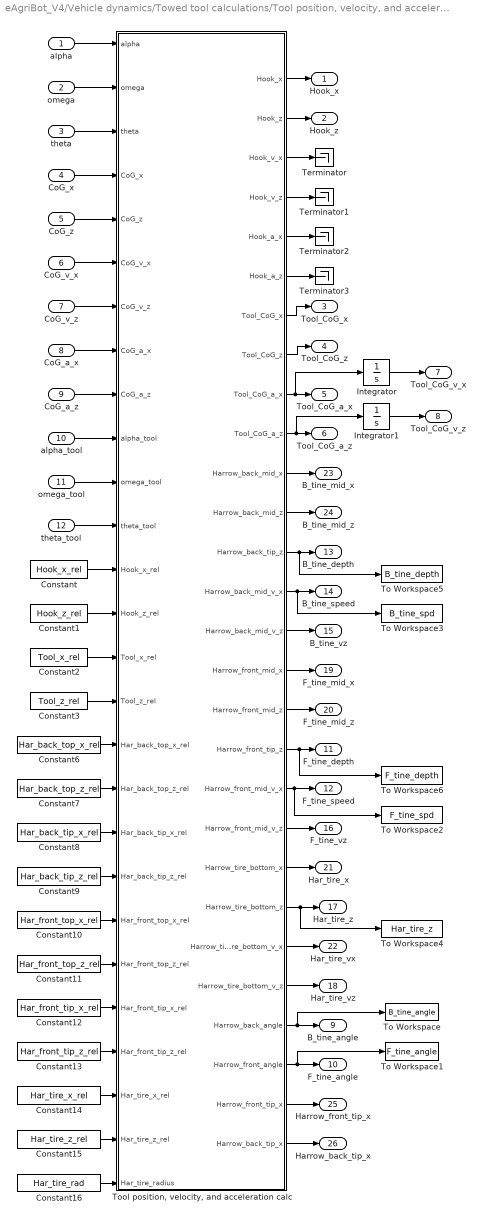
== system eAgriBot_V4/Vehicle dynamics/Towed tool calculations/Tool position, velocity, and acceleration calc ==
  alpha : Inport
  omega : Inport  Port=2
  theta : Inport  Port=3
  CoG_x : Inport  Port=4
  CoG_z : Inport  Port=5
  CoG_v_x : Inport  Port=6
  CoG_v_z : Inport  Port=7
  CoG_a_x : Inport  Port=8
  CoG_a_z : Inport  Port=9
  alpha_tool : Inport  Port=10
  omega_tool : Inport  Port=11
  theta_tool : Inport  Port=12
  Constant : Constant  Value=Hook_x_rel
  Constant1 : Constant  Value=Hook_z_rel
  Constant10 : Constant  Value=Har_front_top_x_rel
  Constant11 : Constant  Value=Har_front_top_z_rel
  Constant12 : Constant  Value=Har_front_tip_x_rel
  Constant13 : Constant  Value=Har_front_tip_z_rel
  Constant14 : Constant  Value=Har_tire_x_rel
  Constant15 : Constant  Value=Har_tire_z_rel
  Constant16 : Constant  Value=Har_tire_rad
  Constant2 : Constant  Value=Tool_x_rel
  Constant3 : Constant  Value=Tool_z_rel
  Constant6 : Constant  Value=Har_back_top_x_rel
  Constant7 : Constant  Value=Har_back_top_z_rel
  Constant8 : Constant  Value=Har_back_tip_x_rel
  Constant9 : Constant  Value=Har_back_tip_z_rel
  Integrator : Integrator
  Integrator1 : Integrator
  Terminator{,1..3} (4 alike) : Terminator
  To Workspace : ToWorkspace  VariableName=B_tine_angle  SaveFormat=Timeseries  SampleTime=-1
  To Workspace1 : ToWorkspace  VariableName=F_tine_angle  SaveFormat=Timeseries  SampleTime=-1
  To Workspace2 : ToWorkspace  VariableName=F_tine_spd  SaveFormat=Timeseries  SampleTime=-1
  To Workspace3 : ToWorkspace  VariableName=B_tine_spd  SaveFormat=Timeseries  SampleTime=-1
  To Workspace4 : ToWorkspace  VariableName=Har_tire_z  SaveFormat=Timeseries  SampleTime=-1
  To Workspace5 : ToWorkspace  VariableName=B_tine_depth  SaveFormat=Timeseries  SampleTime=-1
  To Workspace6 : ToWorkspace  VariableName=F_tine_depth  SaveFormat=Timeseries  SampleTime=-1
  "Tool position, velocity, and acceleration calc" : MATLAB Function  TreatAsAtomicUnit=on  SystemSampleTime=step_size
      settings: MinAlgLoopOccurrences=on
  Hook_x : Outport
  Hook_z : Outport  Port=2
  Tool_CoG_x : Outport  Port=3
  Tool_CoG_z : Outport  Port=4
  Tool_CoG_a_x : Outport  Port=5
  Tool_CoG_a_z : Outport  Port=6
  Tool_CoG_v_x : Outport  Port=7
  Tool_CoG_v_z : Outport  Port=8
  B_tine_angle : Outport  Port=9
  F_tine_angle : Outport  Port=10
  F_tine_depth : Outport  Port=11
  F_tine_speed : Outport  Port=12
  B_tine_depth : Outport  Port=13
  B_tine_speed : Outport  Port=14
  B_tine_vz : Outport  Port=15
  F_tine_vz : Outport  Port=16
  Har_tire_z : Outport  Port=17
  Har_tire_vz : Outport  Port=18
  F_tine_mid_x : Outport  Port=19
  F_tine_mid_z : Outport  Port=20
  Har_tire_x : Outport  Port=21
  Har_tire_vx : Outport  Port=22
  B_tine_mid_x : Outport  Port=23
  B_tine_mid_z : Outport  Port=24
  Harrow_front_tip_x : Outport  Port=25
  Harrow_back_tip_x : Outport  Port=26
  wires:
  alpha_tool/1 -> "Tool position, velocity, and acceleration calc"/10(alpha_tool)
  CoG_z/1 -> "Tool position, velocity, and acceleration calc"/5(CoG_z)
  Constant1/1 -> "Tool position, velocity, and acceleration calc"/14(Hook_z_rel)
  omega_tool/1 -> "Tool position, velocity, and acceleration calc"/11(omega_tool)
  alpha/1 -> "Tool position, velocity, and acceleration calc"/1(alpha)
  CoG_x/1 -> "Tool position, velocity, and acceleration calc"/4(CoG_x)
  CoG_v_z/1 -> "Tool position, velocity, and acceleration calc"/7(CoG_v_z)
  Constant/1 -> "Tool position, velocity, and acceleration calc"/13(Hook_x_rel)
  "Tool position, velocity, and acceleration calc"/10(Tool_CoG_a_z) -> Integrator1/1, Tool_CoG_a_z/1
  "Tool position, velocity, and acceleration calc"/7(Tool_CoG_x) -> Tool_CoG_x/1
  theta/1 -> "Tool position, velocity, and acceleration calc"/3(theta)
  CoG_v_x/1 -> "Tool position, velocity, and acceleration calc"/6(CoG_v_x)
  "Tool position, velocity, and acceleration calc"/9(Tool_CoG_a_x) -> Integrator/1, Tool_CoG_a_x/1
  Constant2/1 -> "Tool position, velocity, and acceleration calc"/15(Tool_x_rel)
  Constant3/1 -> "Tool position, velocity, and acceleration calc"/16(Tool_z_rel)
  omega/1 -> "Tool position, velocity, and acceleration calc"/2(omega)
  theta_tool/1 -> "Tool position, velocity, and acceleration calc"/12(theta_tool)
  "Tool position, velocity, and acceleration calc"/8(Tool_CoG_z) -> Tool_CoG_z/1
  "Tool position, velocity, and acceleration calc"/1(Hook_x) -> Hook_x/1
  "Tool position, velocity, and acceleration calc"/2(Hook_z) -> Hook_z/1
  "Tool position, velocity, and acceleration calc"/3(Hook_v_x) -> Terminator/1
  "Tool position, velocity, and acceleration calc"/4(Hook_v_z) -> Terminator1/1
  "Tool position, velocity, and acceleration calc"/5(Hook_a_x) -> Terminator2/1
  "Tool position, velocity, and acceleration calc"/6(Hook_a_z) -> Terminator3/1
  CoG_a_x/1 -> "Tool position, velocity, and acceleration calc"/8(CoG_a_x)
  CoG_a_z/1 -> "Tool position, velocity, and acceleration calc"/9(CoG_a_z)
  Constant6/1 -> "Tool position, velocity, and acceleration calc"/17(Har_back_top_x_rel)
  Constant7/1 -> "Tool position, velocity, and acceleration calc"/18(Har_back_top_z_rel)
  Constant8/1 -> "Tool position, velocity, and acceleration calc"/19(Har_back_tip_x_rel)
  Constant9/1 -> "Tool position, velocity, and acceleration calc"/20(Har_back_tip_z_rel)
  Constant10/1 -> "Tool position, velocity, and acceleration calc"/21(Har_front_top_x_rel)
  Constant11/1 -> "Tool position, velocity, and acceleration calc"/22(Har_front_top_z_rel)
  Constant12/1 -> "Tool position, velocity, and acceleration calc"/23(Har_front_tip_x_rel)
  Constant14/1 -> "Tool position, velocity, and acceleration calc"/25(Har_tire_x_rel)
  Constant13/1 -> "Tool position, velocity, and acceleration calc"/24(Har_front_tip_z_rel)
  Constant15/1 -> "Tool position, velocity, and acceleration calc"/26(Har_tire_z_rel)
  Constant16/1 -> "Tool position, velocity, and acceleration calc"/27(Har_tire_radius)
  "Tool position, velocity, and acceleration calc"/25(Harrow_back_angle) -> To Workspace/1, B_tine_angle/1
  "Tool position, velocity, and acceleration calc"/26(Harrow_front_angle) -> To Workspace1/1, F_tine_angle/1
  "Tool position, velocity, and acceleration calc"/18(Harrow_front_tip_z) -> To Workspace6/1, F_tine_depth/1
  "Tool position, velocity, and acceleration calc"/19(Harrow_front_mid_v_x) -> To Workspace2/1, F_tine_speed/1
  "Tool position, velocity, and acceleration calc"/13(Harrow_back_tip_z) -> To Workspace5/1, B_tine_depth/1
  "Tool position, velocity, and acceleration calc"/14(Harrow_back_mid_v_x) -> To Workspace3/1, B_tine_speed/1
  "Tool position, velocity, and acceleration calc"/15(Harrow_back_mid_v_z) -> B_tine_vz/1
  "Tool position, velocity, and acceleration calc"/20(Harrow_front_mid_v_z) -> F_tine_vz/1
  "Tool position, velocity, and acceleration calc"/22(Harrow_tire_bottom_z) -> To Workspace4/1, Har_tire_z/1
  "Tool position, velocity, and acceleration calc"/24(Harrow_tire_bottom_v_z) -> Har_tire_vz/1
  "Tool position, velocity, and acceleration calc"/16(Harrow_front_mid_x) -> F_tine_mid_x/1
  "Tool position, velocity, and acceleration calc"/17(Harrow_front_mid_z) -> F_tine_mid_z/1
  "Tool position, velocity, and acceleration calc"/21(Harrow_tire_bottom_x) -> Har_tire_x/1
  "Tool position, velocity, and acceleration calc"/23(Harrow_tire_bottom_v_x) -> Har_tire_vx/1
  "Tool position, velocity, and acceleration calc"/11(Harrow_back_mid_x) -> B_tine_mid_x/1
  "Tool position, velocity, and acceleration calc"/12(Harrow_back_mid_z) -> B_tine_mid_z/1
  Integrator/1 -> Tool_CoG_v_x/1
  Integrator1/1 -> Tool_CoG_v_z/1
  "Tool position, velocity, and acceleration calc"/27(Harrow_front_tip_x) -> Harrow_front_tip_x/1
  "Tool position, velocity, and acceleration calc"/28(Harrow_back_tip_x) -> Harrow_back_tip_x/1

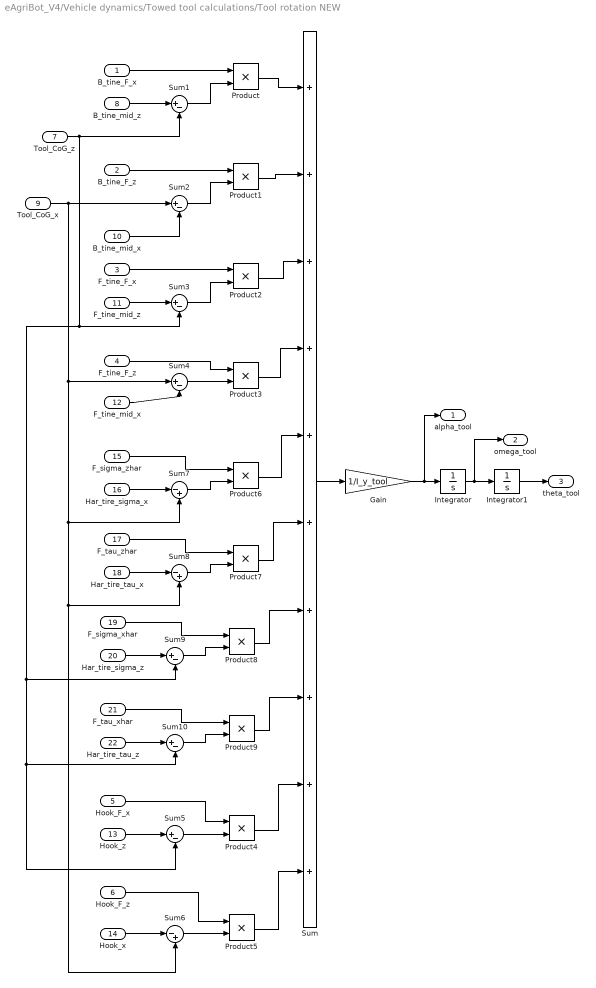
== system eAgriBot_V4/Vehicle dynamics/Towed tool calculations/Tool rotation NEW ==
  B_tine_F_x : Inport
  B_tine_F_z : Inport  Port=2
  F_tine_F_x : Inport  Port=3
  F_tine_F_z : Inport  Port=4
  Hook_F_x : Inport  Port=5
  Hook_F_z : Inport  Port=6
  Tool_CoG_z : Inport  Port=7
  B_tine_mid_z : Inport  Port=8
  Tool_CoG_x : Inport  Port=9
  B_tine_mid_x : Inport  Port=10
  F_tine_mid_z : Inport  Port=11
  F_tine_mid_x : Inport  Port=12
  Hook_z : Inport  Port=13
  Hook_x : Inport  Port=14
  F_sigma_zhar : Inport  Port=15
  Har_tire_sigma_x : Inport  Port=16
  F_tau_zhar : Inport  Port=17
  Har_tire_tau_x : Inport  Port=18
  F_sigma_xhar : Inport  Port=19
  Har_tire_sigma_z : Inport  Port=20
  F_tau_xhar : Inport  Port=21
  Har_tire_tau_z : Inport  Port=22
  Gain : Gain  Gain=1/I_y_tool
  Integrator : Integrator  InitialCondition=omega_tool_init
  Integrator1 : Integrator  InitialCondition=theta_tool_init
  Product{,1..9} (10 alike) : Product
  Sum : Sum  Inputs=++++++++++
  Sum{1..5,9..10} (7 alike) : Sum  Inputs=|+-
  Sum6 : Sum  Inputs=|-+
  Sum7 : Sum  Inputs=|-+
  Sum8 : Sum  Inputs=|-+
  alpha_tool : Outport
  omega_tool : Outport  Port=2
  theta_tool : Outport  Port=3
  wires:
  B_tine_F_x/1 -> Product/1
  B_tine_mid_z/1 -> Sum1/1
  Tool_CoG_z/1 -> Sum3/2, Sum10/2, Sum5/2, Sum9/2, Sum1/2
  Sum1/1 -> Product/2
  Product/1 -> Sum/1
  Integrator1/1 -> theta_tool/1
  Gain/1 -> alpha_tool/1, Integrator/1
  Integrator/1 -> omega_tool/1, Integrator1/1
  Sum/1 -> Gain/1
  B_tine_mid_x/1 -> Sum2/2
  B_tine_F_z/1 -> Product1/1
  Sum2/1 -> Product1/2
  Product1/1 -> Sum/2
  F_tine_F_x/1 -> Product2/1
  F_tine_mid_z/1 -> Sum3/1
  Sum3/1 -> Product2/2
  Product2/1 -> Sum/3
  F_tine_F_z/1 -> Product3/1
  F_tine_mid_x/1 -> Sum4/2
  Sum4/1 -> Product3/2
  Product3/1 -> Sum/4
  Hook_F_x/1 -> Product4/1
  Sum5/1 -> Product4/2
  Hook_z/1 -> Sum5/1
  Hook_F_z/1 -> Product5/1
  Sum6/1 -> Product5/2
  Hook_x/1 -> Sum6/1
  Product6/1 -> Sum/5
  F_sigma_zhar/1 -> Product6/1
  Har_tire_sigma_x/1 -> Sum7/1
  Sum7/1 -> Product6/2
  Har_tire_tau_x/1 -> Sum8/1
  F_tau_zhar/1 -> Product7/1
  Tool_CoG_x/1 -> Sum2/1, Sum7/2, Sum8/2, Sum6/2, Sum4/1
  Sum8/1 -> Product7/2
  Product7/1 -> Sum/6
  Har_tire_sigma_z/1 -> Sum9/1
  F_sigma_xhar/1 -> Product8/1
  Sum9/1 -> Product8/2
  Product8/1 -> Sum/7
  Product5/1 -> Sum/10
  Product4/1 -> Sum/9
  Har_tire_tau_z/1 -> Sum10/1
  Product9/1 -> Sum/8
  F_tau_xhar/1 -> Product9/1
  Sum10/1 -> Product9/2
